simulink subsystem "Speed_Calc_FastSlow"  (R2022b)
settings: Solver=VariableStepAuto  StartTime=0.0  StopTime=10.0  RelTol=1e-3
undefined symbols (not defined in the file): CounterFactor_us
libraries: simulink x1
settings Model: Creator=unix  LastModifiedBy=unix

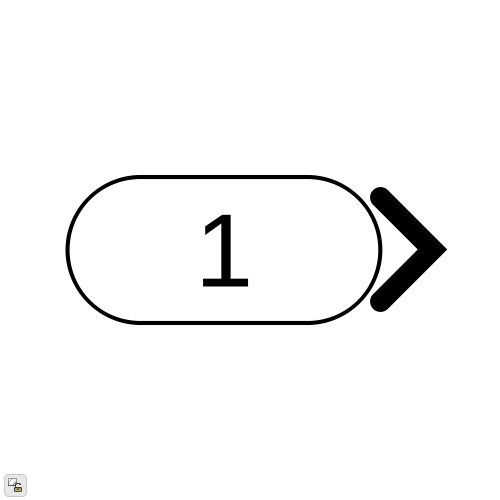
[thumbnail: Simulink's stored preview of the top-level diagram]
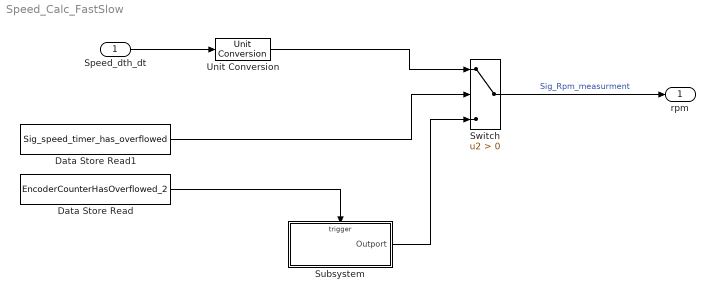
== system Speed_Calc_FastSlow ==
  Speed_dth_dt : Inport
  Data Store Read : DataStoreRead  DataStoreName=EncoderCounterHasOverflowed_2  IndexOptions=Index vector (dialog)  Indices=1  OutputSizes=1
  Data Store Read1 : DataStoreRead  DataStoreName=Sig_speed_timer_has_overflowed  IndexOptions=Index vector (dialog)  Indices=1  OutputSizes=1
  Subsystem : Subsystem
  Switch : Switch  Criteria=u2 > Threshold  SaturateOnIntegerOverflow=off  InputSameDT=off
  Unit Conversion : UnitConversion
  rpm : Outport
  wires:
  Speed_dth_dt/1 -> Unit Conversion/1
  Data Store Read1/1 -> Switch/2
  Data Store Read/1 -> Subsystem/Trigger
  Subsystem/1(Outport) -> Switch/3
  Switch/1 -> rpm/1  "Sig_Rpm_measurment"
  Unit Conversion/1 -> Switch/1

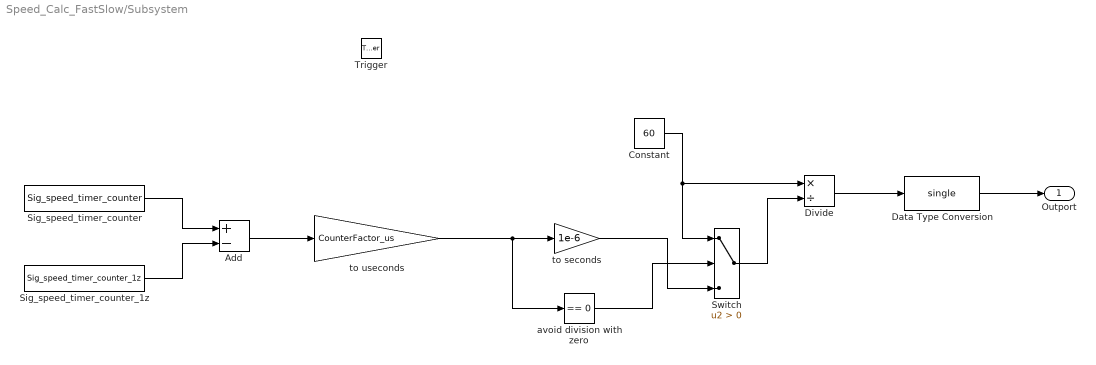
== system Speed_Calc_FastSlow/Subsystem ==
  Trigger : TriggerPort  VariantControl=(inherit)  PortDimensions=1
  Add : Sum  Inputs=+-
  Constant : Constant  Value=60  OutDataTypeStr=uint8
  Data Type Conversion : DataTypeConversion  OutDataTypeStr=single  SaturateOnIntegerOverflow=off  RndMeth=Floor
  Divide : Product  Inputs=*/  SaturateOnIntegerOverflow=on
  Sig_speed_timer_counter : DataStoreRead  DataStoreName=Sig_speed_timer_counter  IndexOptions=Index vector (dialog)  Indices=1  OutputSizes=1
  Sig_speed_timer_counter_1z : DataStoreRead  DataStoreName=Sig_speed_timer_counter_1z  IndexOptions=Index vector (dialog)  Indices=1  OutputSizes=1
  Switch : Switch  Criteria=u2 > Threshold  SaturateOnIntegerOverflow=off  InputSameDT=off
  avoid division with zero : simulink/Logic and Bit Operations/Compare To Zero  relop===  OutDataTypeStr=boolean
  to seconds : Gain  Gain=1e-6  ParamDataTypeStr=single  OutDataTypeStr=fixdt(0,16,2^-16,0)
  to useconds : Gain  Gain=CounterFactor_us  ParamDataTypeStr=fixdt(0,16,2^0,500)
  Outport : Outport
  wires:
  Data Type Conversion/1 -> Outport/1
  Divide/1 -> Data Type Conversion/1
  avoid division with zero/1 -> Switch/2
  Switch/1 -> Divide/2
  to seconds/1 -> Switch/3
  Constant/1 -> Divide/1, Switch/1
  to useconds/1 -> to seconds/1, avoid division with zero/1
  Add/1 -> to useconds/1
  Sig_speed_timer_counter/1 -> Add/1
  Sig_speed_timer_counter_1z/1 -> Add/2
